simulink model "Lotka_Volterra"  (R2021a)
settings: Solver=ode15s  StartTime=0.0  StopTime=10.0  FixedStep=0.1  RelTol=1e-3  EnableMultiTasking=on
libraries: hwlogiciolib x1
settings Model: Creator=acalame  LastModifiedBy=alvic
settings SolverCC: AlgebraicLoopSolver=TrustRegion  AutoInsertRateTranBlk=on
settings DataIOCC: LimitDataPoints=on
settings OptimizationCC: LifeSpan=inf
settings DebuggingCC: AllowSymbolicDim=off  SFUnexpectedBacktrackingDiag=warning  SFNoUnconditionalDefaultTransitionDiag=warning  SFExecutionAtInitializationDiag=none  ArithmeticOperatorsInVariantConditions=warning
settings SFSimCC: SimUseLocalCustomCode=off  CustomCodeUndefinedFunction=UseInterfaceOnly
settings RTWCC: RTWUseLocalCustomCode=off
settings CodeAppCC: StateflowObjectComments=on
settings GRTTargetCC: TargetLangStandard=C89/C90 (ANSI)
settings ConfigComp: CovMetricSettings=dw  CovSaveCumulativeToWorkspaceVar=on  CovSaveSingleToWorkspaceVar=on  CovExternalEMLEnable=off  CovSFcnEnable=off

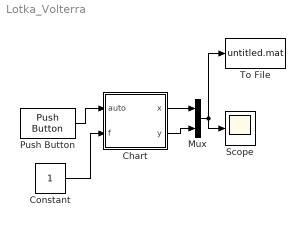
== system Lotka_Volterra ==
  Chart : Stateflow chart  TreatAsAtomicUnit=on
  Constant : Constant
  Mux : Mux  Inputs=2
  Push Button : hwlogiciolib/Push Button  SimMode=Dialog  NumHMI=1  PB1=Off  PB2=Off  PB3=Off  PB4=Off  PB5=Off  PB6=Off  PB7=Off  PB8=Off  HMISampleTime=-1  HMIKind=pushbuttons  HMILabel=PB  LastTargetBoard=None
      settings: SourceProductBaseCode=HW
  Scope : Scope
  To File : ToFile  SaveFormat=Timeseries
  wires:
  Chart/1(x) -> Mux/1
  Chart/2(y) -> Mux/2
  Push Button/1 -> Chart/1(auto)
  Constant/1 -> Chart/2(f)
  Mux/1 -> Scope/1, To File/1

== stateflow chart Lotka_Volterra/Chart ==
  settings: updateMethod=CONTINUOUS
  state evolution_de_requin_et_sardine
    during :
    x_dot = a*x - b*x*y;
    y_dot =  c*x*y - d*y;
  state evolution_de_requin_et_sardine_peche
    during :
    x_dot = a*x - b*x*y - f*x;
    y_dot =  c*x*y - d*y;
  (default) -> evolution_de_requin_et_sardine : {x=3.33, y = 4}
  evolution_de_requin_et_sardine -> evolution_de_requin_et_sardine_peche : [x>xmax && auto == true]
  evolution_de_requin_et_sardine_peche -> evolution_de_requin_et_sardine : [x<xmin]
  data: a local =2; b local =1; x output =3.33; y output =4; d local =1; c local =0.3; xmax local =3.4; xmin local =3.2; auto input boolean; f input =1
  data x settings: updateMethod=SF_CONTINUOUS_TIME_DATA
  data y settings: updateMethod=SF_CONTINUOUS_TIME_DATA
